simulink model "full_step"  (R2021b)
settings: Solver=FixedStepDiscrete  StartTime=0.0  StopTime=inf  FixedStep=1e-4  RelTol=1e-3
libraries: dspsigops x4, simulink_extras x3, speedgoatlib_IO102 x2
settings Model: Creator=wasynczu  LastModifiedBy=wasynczu
settings SolverCC: ConcurrentTasks=on  PositivePriorityOrder=on
settings OptimizationCC: BlockReduction=off  OptimizeBlockIOStorage=off
settings DebuggingCC: TasksWithSamePriorityMsg=none
settings HardwareCC: ProdBitPerLong=64  ProdLongLongMode=on  ProdHWDeviceType=Intel->x86-64 (Linux 64)
settings RTWCC: Description=Simulink Real-Time  SystemTargetFile=slrealtime.tlc  TemplateMakefile=slrealtime_default_tmf  Toolchain=Simulink Real-Time Toolchain  BuildConfiguration=Faster Runs  CodeExecutionProfiling=on  TargetLang=C++

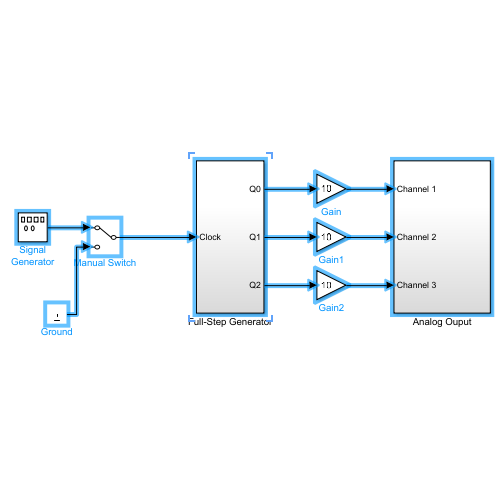
[thumbnail: Simulink's stored preview of the top-level diagram]
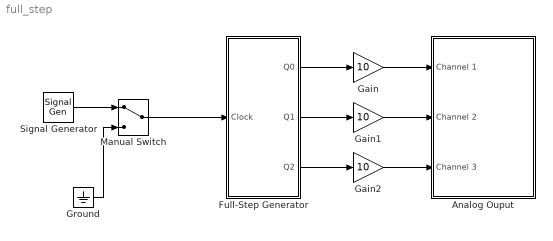
== system full_step ==
  Analog Ouput : Subsystem
  Full-Step Generator : Subsystem
  Gain : Gain  Gain=10
  Gain1 : Gain  Gain=10
  Gain2 : Gain  Gain=10
  Ground : Ground
  Manual Switch : ManualSwitch
  Signal Generator : SignalGenerator  WaveForm=square  Frequency=10
  wires:
  Manual Switch/1 -> Full-Step Generator/1(Clock)
  Signal Generator/1 -> Manual Switch/1
  Ground/1 -> Manual Switch/2
  Full-Step Generator/1(Q0) -> Gain/1
  Full-Step Generator/2(Q1) -> Gain1/1
  Full-Step Generator/3(Q2) -> Gain2/1
  Gain/1 -> Analog Ouput/1(Channel 1)
  Gain2/1 -> Analog Ouput/3(Channel 3)
  Gain1/1 -> Analog Ouput/2(Channel 2)

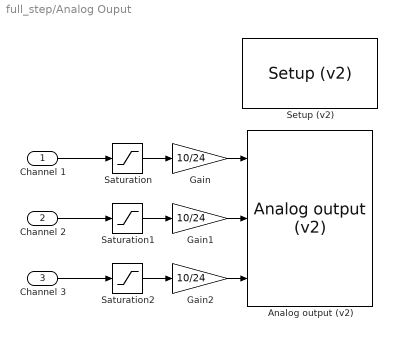
== system full_step/Analog Ouput ==
  Channel 1 : Inport
  Channel 2 : Inport  Port=2
  Channel 3 : Inport  Port=3
  "Analog output (v2) " : speedgoatlib_IO102/Analog output (v2)   id=1  channels=[1 2 3]  range=1  ts=-1  pciSlot=-1
      settings: SourceProductName=Simulink Real-Time: Speedgoat I/O Blockset
  Gain : Gain  Gain=10/24
  Gain1 : Gain  Gain=10/24
  Gain2 : Gain  Gain=10/24
  Saturation : Saturate  UpperLimit=24  LowerLimit=-24
  Saturation1 : Saturate  UpperLimit=24  LowerLimit=-24
  Saturation2 : Saturate  UpperLimit=24  LowerLimit=-24
  "Setup (v2) " : speedgoatlib_IO102/Setup (v2)   id=1  range=+-10V  cal=off  pciSlot=-1  adCoupling=Single-ended  adChannelMode=Multiple-channel (enter number of channels below)  adChannel=4  daChannel=[1,2,3]  daInitValue=[0]  daReset=[1]  DioDirectionLo=Input  DioDirectionHi=Output  doChannel=[9]  doInitValue=[0]  doReset=[1]  diChannel=[1]
      settings: SourceProductName=Simulink Real-Time: Speedgoat I/O Blockset
  wires:
  Saturation/1 -> Gain/1
  Saturation1/1 -> Gain1/1
  Saturation2/1 -> Gain2/1
  Gain1/1 -> "Analog output (v2) "/2
  Gain/1 -> "Analog output (v2) "/1
  Gain2/1 -> "Analog output (v2) "/3
  Channel 2/1 -> Saturation1/1
  Channel 3/1 -> Saturation2/1
  Channel 1/1 -> Saturation/1

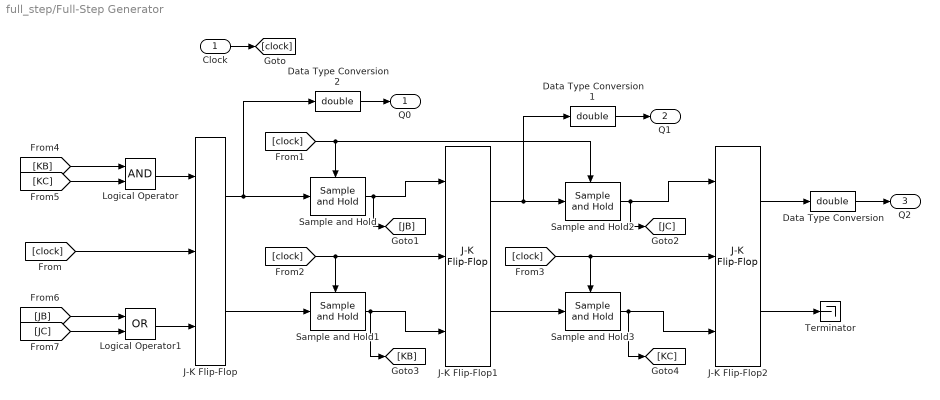
== system full_step/Full-Step Generator ==
  Clock : Inport
  Data Type Conversion : DataTypeConversion  OutDataTypeStr=double
  Data Type Conversion1 : DataTypeConversion  OutDataTypeStr=double
  Data Type Conversion2 : DataTypeConversion  OutDataTypeStr=double
  J-K Flip-Flop : simulink_extras/Flip Flops/J-K Flip-Flop  initial_condition=0
  J-K Flip-Flop1 : simulink_extras/Flip Flops/J-K Flip-Flop  initial_condition=0
  J-K Flip-Flop2 : simulink_extras/Flip Flops/J-K Flip-Flop  initial_condition=0
  Logical Operator : Logic  AllPortsSameDT=off  OutDataTypeStr=boolean
  Logical Operator1 : Logic  Operator=OR  AllPortsSameDT=off  OutDataTypeStr=boolean
  Sample and Hold{,1..3} (4 alike) : dspsigops/Sample and Hold  trig=Rising edge  initCond=0  latchinput=off
  Terminator : Terminator
  Q0 : Outport
  Q1 : Outport  Port=2
  Q2 : Outport  Port=3
  wires:
  Clock/1 -> [clock]
  [clock] -> J-K Flip-Flop/2
  [clock] -> Sample and Hold2/Trigger, Sample and Hold/Trigger
  J-K Flip-Flop/2 -> Sample and Hold1/1
  [clock] -> Sample and Hold1/Trigger, J-K Flip-Flop1/2
  J-K Flip-Flop1/1 -> Data Type Conversion1/1, Sample and Hold2/1
  J-K Flip-Flop1/2 -> Sample and Hold3/1
  Sample and Hold/1 -> [JB], J-K Flip-Flop1/1
  Sample and Hold1/1 -> [KB], J-K Flip-Flop1/3
  [clock] -> J-K Flip-Flop2/2, Sample and Hold3/Trigger
  Sample and Hold3/1 -> [KC], J-K Flip-Flop2/3
  Sample and Hold2/1 -> [JC], J-K Flip-Flop2/1
  J-K Flip-Flop2/1 -> Data Type Conversion/1
  Data Type Conversion/1 -> Q2/1
  Data Type Conversion1/1 -> Q1/1
  J-K Flip-Flop/1 -> Data Type Conversion2/1, Sample and Hold/1
  Data Type Conversion2/1 -> Q0/1
  J-K Flip-Flop2/2 -> Terminator/1
  [KB] -> Logical Operator/1
  [KC] -> Logical Operator/2
  Logical Operator/1 -> J-K Flip-Flop/1
  [JB] -> Logical Operator1/1
  [JC] -> Logical Operator1/2
  Logical Operator1/1 -> J-K Flip-Flop/3
